simulink model "QAM16_adalm_radio_emulation"  (R2024b)
settings: Solver=VariableStepAuto  StartTime=0.0  StopTime=38  RelTol=1e-3
PreLoadFcn:
  | % 16-QAM demo. SJSU. Fall 2020
  | 
  | alpha = 1/2;
  | 
  | Rs = 400000;                     % Sampling rate for radios
  | Nf = 2000;                        % Frame size
  | 
  | Gt = -5;                             % Transmitter radio gain
  | amp = 0.5;                        % Transmited signal amplitude
  | 
  | Gr = 25;                             % Receiver radio gain
  | 
  | Deltaf = 500;                     % Frequency error
  | phi = -pi/6;                        % Phase error
  | 
  | EsNo = 20;
  | var = 10^-(EsNo/10)/2;                   % AWGN power
  | 
  | BarkerCode=[1,1,1,1,1,-1,-1,1,1,-1,1,-1,1];
  | 
  | load(QPSK_radio_parameters.mat)
PostLoadFcn:
  | laod(QPSK_radio_parameters.mat)
undefined symbols (not defined in the file or in its folder): QAM, sdrqpskrx
libraries: commrflib2 x3, commrfcorlib x2, commsync2 x2, commfilt2 x2, simulink x2, dspstat3 x1, commrandsrc3 x1, dspsigops x1, commsequence2 x1, commdigbbndam3 x1
settings Model: Creator=The MathWorks, Inc.  LastModifiedBy=14083
settings SolverCC: AlgebraicLoopSolver=TrustRegion  AutoInsertRateTranBlk=on
settings DataIOCC: LimitDataPoints=on  SaveFormat=Structure  SaveOutput=off  SignalLogging=off  DSMLogging=off  SaveTime=off  ReturnWorkspaceOutputs=off
settings OptimizationCC: DefaultParameterBehavior=Inlined  ExpressionDepthLimit=2147483647  LocalBlockOutputs=off  LifeSpan=inf  SimCompilerOptimization=on
settings DebuggingCC: AlgebraicLoopMsg=error  UnderspecifiedInitializationDetection=Classic  MergeDetectMultiDrivingBlocksExec=none  SolverPrmCheckMsg=warning  SingleTaskRateTransMsg=error  ParameterPrecisionLossMsg=none  FcnCallInpInsideContextMsg=warning  UnconnectedInputMsg=warning  UnconnectedOutputMsg=warning  UnconnectedLineMsg=warning  AllowSymbolicDim=off  StateNameClashWarn=warning  SFUnexpectedBacktrackingDiag=warning  SFNoUnconditionalDefaultTransitionDiag=warning  SFExecutionAtInitializationDiag=none  ArithmeticOperatorsInVariantConditions=warning
settings HardwareCC: ProdBitPerPointer=32  ProdBitPerSizeT=32  ProdBitPerPtrDiffT=32  ProdLargestAtomicFloat=None  ProdIntDivRoundTo=Undefined  ProdEndianess=Unspecified  ProdWordSize=32  ProdHWDeviceType=32-bit Generic  TargetBitPerPointer=64  TargetBitPerSizeT=64  TargetBitPerPtrDiffT=64  TargetLongLongMode=on  TargetIntDivRoundTo=Zero  TargetEndianess=LittleEndian  TargetWordSize=64  TargetHWDeviceType=Generic->MATLAB Host Computer  ProdEqTarget=off
settings ModelReferenceCC: EnableRefExpFcnMdlSchedulingChecks=on  PropagateSignalLabelsOutOfModel=off
settings SFSimCC: SimUseLocalCustomCode=off  CustomCodeUndefinedFunction=UseInterfaceOnly
settings RTWCC: RTWUseLocalCustomCode=off  GPUComputeCapability=3.5
settings RTWCC: CustomSourceCode=|
  | #include <stdio.h>
  | #include <stdlib.h>
settings CodeAppCC: StateflowObjectComments=on
settings GRTTargetCC: TargetLangStandard=C89/C90 (ANSI)  CombineOutputUpdateFcns=off  GRTInterface=on
settings ConfigComp: CovMetricSettings=dw  CovSaveCumulativeToWorkspaceVar=on  CovSaveSingleToWorkspaceVar=on  CovExternalEMLEnable=off  CovSFcnEnable=off

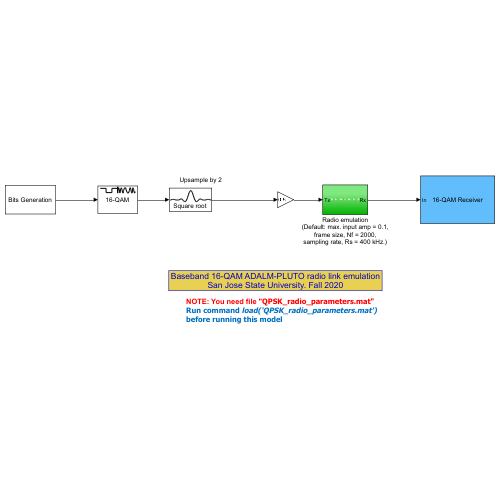
[thumbnail: Simulink's stored preview of the top-level diagram]
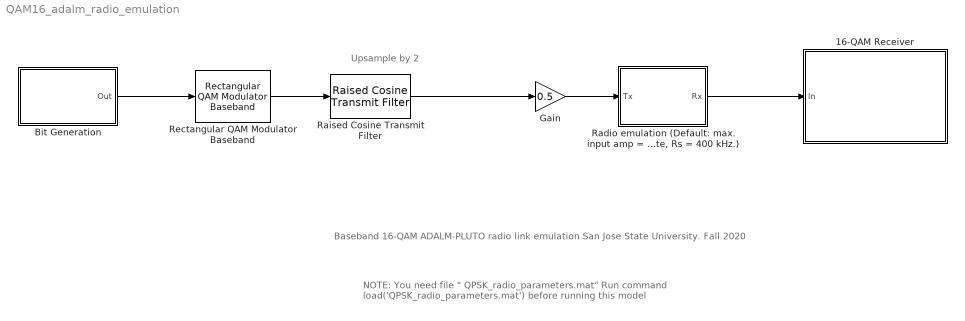
== system QAM16_adalm_radio_emulation ==
  note: NOTE: You need file " QPSK_radio_parameters.mat"
      | Run command load('QPSK_radio_parameters.mat') before running this model
  note: Upsample by 2
  note: Baseband 16-QAM ADALM-PLUTO radio link emulation
      | San Jose State University. Fall 2020
  16-QAM Receiver : Subsystem
      mask Display: disp('16-QAM Receiver')
  Bit Generation : Subsystem
      mask Display: disp('Bits Generation')
  Gain : Gain  Gain=0.5
  "Radio emulation (Default: max. input amp = 0.1, frame size, Nf = 2000, sampling rate, Rs = 400 kHz.)" : Subsystem
  Raised Cosine Transmit Filter : commfilt2/Raised Cosine Transmit Filter  filtType=Square root  R=alpha  filtSpan=10  N=2  filterGain=1  InputProcessing=Columns as channels (frame based)  RateOptions=Enforce single-rate processing  framing=Mute  checkCoeff=off  variableName=rcTxFilt1  checkGain=Normalized  sampMode=Mute  saveAsFlag=0  currentFiltSpan=10  D=5  launchFVT=on  roundingMode=Floor  overflowMode=off  coeffDataTypeStr=Inherit: Same word length as input  coeffMin=[]  coeffMax=[]  coeffLastDataTypeStr=Inherit: Same word length as input  outputDataTypeStr=Inherit: Same as accumulator  outputMin=[]  outputMax=[]  outputLastDataTypeStr=Inherit: Same as accumulator
  Rectangular QAM Modulator Baseband : commdigbbndam3/Rectangular QAM Modulator Baseband  M=16  InType=Bit  Enc=Gray  Mapping=[0:15]  PowType=Average Power  MinDist=2  AvgPow=1  PeakPow=1  Ph=0  outDtype=double  outWordLen=16  outUDDataType=sfix(16)  outFracLenMode=Best precision  outFracLen=15  outDataTypeStr=double  outLastDataTypeStr=double
  wires:
  Bit Generation/1(Out) -> Rectangular QAM Modulator Baseband/1
  "Radio emulation (Default: max. input amp = 0.1, frame size, Nf = 2000, sampling rate, Rs = 400 kHz.)"/1(Rx) -> 16-QAM Receiver/1(In)
  Rectangular QAM Modulator Baseband/1 -> Raised Cosine Transmit Filter/1
  Gain/1 -> "Radio emulation (Default: max. input amp = 0.1, frame size, Nf = 2000, sampling rate, Rs = 400 kHz.)"/1(Tx)
  Raised Cosine Transmit Filter/1 -> Gain/1

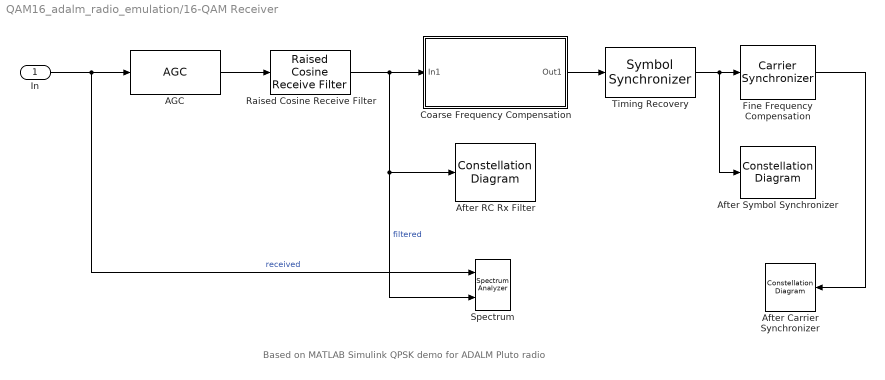
== system QAM16_adalm_radio_emulation/16-QAM Receiver ==
  note: Based on MATLAB Simulink QPSK demo for ADALM Pluto radio
  In : Inport
  AGC : commrfcorlib/AGC  LegacyMode=off  DetectorMethod=Rectifier  LoopMethod=Linear  UpdatePeriod=100  StepSize=0.1  AdaptationStepSize=0.01  DesiredOutputPower=1  AveragingLength=sdrqpskrx.AveragingLength  MaximumGain=30  MaxPowerGain=sdrqpskrx.MaxPowerGain  GainOutputPort=off  InputPowerOutputPort=off  SimulateUsing=Code generation
  After Carrier Synchronizer : ConstellationDiagram  Tag=ScatterPlot  WindowPosition=[1063.000000,378.000000,414.000000,420.000000,]  Visible=on  ScopeFrameLocation=window  SamplesPerSymbol=sdrqpskrx.Interpolation  SymbolsToDisplaySource=Property  SymbolsToDisplay=sdrqpskrx.FrameSize  ReferenceConstellation=16-QAM  Title=After Carrier Synchronizer  XLimits=[-3.25,3.25]  YLimits=[-2.8 2.8]  ShowReferenceConstellation=off  ColorFading=on  DefaultConfigurationName=comm.scopes.ConstellationDiagramBlockCfg
  After RC Rx Filter : ConstellationDiagram  Tag=ScatterPlot  WindowPosition=[218.000000,376.000000,414.000000,423.000000,]  Visible=on  ScopeFrameLocation=window  SamplesPerSymbol=sdrqpskrx.Interpolation  SymbolsToDisplaySource=Property  SymbolsToDisplay=sdrqpskrx.FrameSize  ReferenceConstellation=16-QAM  Title=After Raised Cosine Rx Filter  XLimits=[-2.6623352812286596,2.6684400675627136]  YLimits=[-2.6508250238276854,2.7130991397079955]  ShowReferenceConstellation=off  ColorFading=on  DefaultConfigurationName=comm.scopes.ConstellationDiagramBlockCfg
  After Symbol Synchronizer : ConstellationDiagram  Tag=ScatterPlot  WindowPosition=[633.000000,376.000000,432.000000,422.000000,]  Visible=on  ScopeFrameLocation=window  SamplesPerSymbol=2  SymbolsToDisplaySource=Property  SymbolsToDisplay=sdrqpskrx.FrameSize  ReferenceConstellation=QPSK  Title=After Symbol Synchronizer  XLimits=[-3.4,3.4]  YLimits=[-2.8 2.8]  ShowReferenceConstellation=off  ColorFading=on  DefaultConfigurationName=comm.scopes.ConstellationDiagramBlockCfg
  Coarse Frequency Compensation : Subsystem
      mask Display: fprintf('Coarse Frequency\nCompensation')
  Fine Frequency Compensation : commsync2/Carrier Synchronizer  Modulation=QAM  ModulationPhaseOffset=Auto  CustomPhaseOffset=0  SamplesPerSymbol=sdrqpskrx.Interpolation/sdrqpskrx.Decimation  DampingFactor=1  NormalizedLoopBandwidth=0.01  EstimatedPhaseErrorOutputPort=off  SimulateUsing=Code generation
  Raised Cosine Receive Filter : commfilt2/Raised Cosine Receive Filter  filtType=Square root  R=alpha  filtSpan=sdrqpskrx.RaisedCosineFilterSpan  N=sdrqpskrx.Interpolation  downFactor=sdrqpskrx.Decimation  downOffset=0  filterGain=1  InputProcessing=Columns as channels (frame based)  RateOptions=Enforce single-rate processing  framing=Mute  checkCoeff=off  variableName=rcRxFilt  currentFiltSpan=10  D=5  inputOffset=0  sampMode=Mute  saveAsFlag=0  rateMode=Downsampling  checkGain=Normalized  launchFVT=on  roundingMode=Floor  overflowMode=off  coeffDataTypeStr=Inherit: Same word length as input  coeffMin=[]  coeffMax=[]  coeffLastDataTypeStr=Inherit: Same word length as input  accumDataTypeStr=Inherit: Same as product output  accumLastDataTypeStr=Inherit: Same as product output  outputDataTypeStr=Inherit: Same as accumulator  outputMin=[]  outputMax=[]  outputLastDataTypeStr=Inherit: Same as accumulator
  Spectrum : SpectrumAnalyzer  NumInputPorts=2  WindowPosition=[27.000000,20.000000,800.000000,364.000000,]  Visible=on  ScopeFrameLocation=window  Method=Welch  SampleRate=100654.15132949  AxesScaling=Manual  RBWSource=Property  RBW=75  FFTLength=128  Span=100000  StartFrequency=-50000  StopFrequency=50000  AveragingMethod=Running  SpectralAverages=2  SpectrumUnits=dBW  Title=Before and After Raised Cosine Rx Filter  YLabel=Power Spectrum  YLimits=[-137.6344738236879266,40]  ShowLegend=on  AllowFFTLengthLessThanSamplesPerUpdate=on  DefaultConfigurationName=spbscopes.SpectrumAnalyzerBlockCfg  IsFrequencyInputMode=0  FrequencyVectorPort=0  FrequencyVectorFromPort=0  FrequencyInputRBWPort=0  FrequencyInputRBWFromPort=0
  Timing Recovery : commsync2/Symbol Synchronizer  Modulation=PAM/PSK/QAM  TimingErrorDetector=Gardner (non-data-aided)  SamplesPerSymbol=sdrqpskrx.Interpolation/sdrqpskrx.Decimation  DampingFactor=1  NormalizedLoopBandwidth=0.01  DetectorGain=sdrqpskrx.TimingErrorDetectorGain  TimingErrorOutputPort=off  SimulateUsing=Code generation
  wires:
  Raised Cosine Receive Filter/1 -> Coarse Frequency Compensation/1(In1), Spectrum/2, After RC Rx Filter/1  "filtered"
  Coarse Frequency Compensation/1(Out1) -> Timing Recovery/1
  AGC/1 -> Raised Cosine Receive Filter/1
  Fine Frequency Compensation/1 -> After Carrier Synchronizer/1
  Timing Recovery/1 -> Fine Frequency Compensation/1, After Symbol Synchronizer/1
  In/1 -> Spectrum/1, AGC/1  "received"

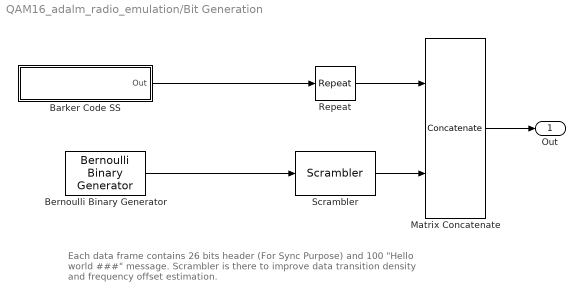
== system QAM16_adalm_radio_emulation/Bit Generation ==
  note: Each data frame contains 26 bits header (For Sync Purpose) and 100
      | "Hello world ###" message. Scrambler is there to improve data
      | transition density and frequency offset estimation.
  Barker Code SS : Subsystem
      mask Display: disp('Unipolar\nBarker Code')
  Bernoulli Binary Generator : commrandsrc3/Bernoulli Binary Generator  ProbabilityOfZero=0.5  SeedSource=Auto  Seed=0  SampleTime=1/200000  SamplesPerFrame=100*40-13*2  OutputDataType=double  SimulateUsing=Interpreted execution
  Matrix Concatenate : Concatenate  Mode=Multidimensional array
  Repeat : dspsigops/Repeat  FactorSource=Dialog parameter  N=2  Nmax=16  InputProcessing=Columns as channels (frame based)  RateOptions=Enforce single-rate processing  ic=0  mode=Unused parameter value
  Scrambler : commsequence2/Scrambler  M=2  poly=[1 1 1 0 1]  iniStaSource=Dialog Parameter  ini_sta=[0 0 0 0]  resetViaPort=off
  Out : Outport  VectorParamsAs1DForOutWhenUnconnected=off
  wires:
  Barker Code SS/1(Out) -> Repeat/1
  Matrix Concatenate/1 -> Out/1
  Repeat/1 -> Matrix Concatenate/1
  Scrambler/1 -> Matrix Concatenate/2
  Bernoulli Binary Generator/1 -> Scrambler/1

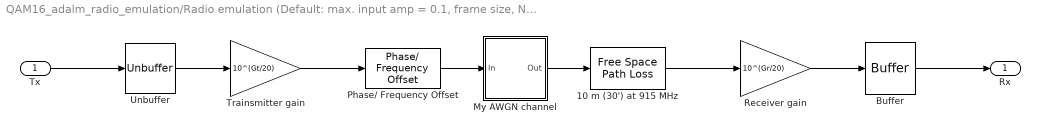
== system QAM16_adalm_radio_emulation/Radio emulation (Default: max. input amp = 0.1, frame size, Nf = 2000, sampling rate, Rs = 400 kHz.) ==
  Tx : Inport
  10 m (30') at 915 MHz : commrflib2/Free Space Path Loss  mode=Distance and Frequency  dB=10  d=10/1000  fc=915
  Buffer : Buffer  N=Nf  OutputFrames=off
  My AWGN channel : Subsystem
  Phase/ Frequency Offset : commrflib2/Phase// Frequency Offset  phaseOffset=phi  freqPort=off  freqOffset=Deltaf
  Receiver gain : Gain  Gain=10^(Gr/20)
  Trainsmitter gain : Gain  Gain=10^(Gt/20)
  Unbuffer : Unbuffer
  Rx : Outport
  wires:
  Tx/1 -> Unbuffer/1
  My AWGN channel/1(Out) -> 10 m (30') at 915 MHz/1
  Phase/ Frequency Offset/1 -> My AWGN channel/1(In)
  10 m (30') at 915 MHz/1 -> Receiver gain/1
  Receiver gain/1 -> Buffer/1
  Unbuffer/1 -> Trainsmitter gain/1
  Buffer/1 -> Rx/1
  Trainsmitter gain/1 -> Phase/ Frequency Offset/1

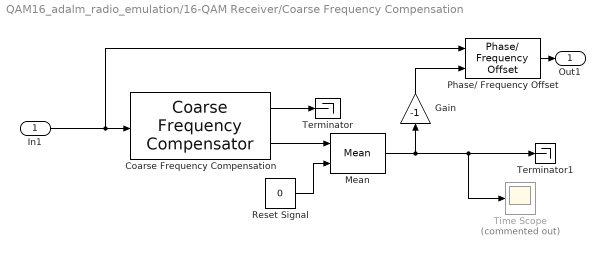
== system QAM16_adalm_radio_emulation/16-QAM Receiver/Coarse Frequency Compensation ==
  In1 : Inport
  Coarse Frequency Compensation : commrfcorlib/Coarse Frequency Compensator  Modulation=QPSK  Algorithm=Correlation-based  FrequencyResolution=25  MaximumFrequencyOffset=12.5e3  SamplesPerSymbol=4  EstimatedFreqOffsetPort=on  SimulateUsing=Code generation
  Gain : Gain  Gain=-1
  Mean : dspstat3/Mean  run=on  InputProcessing=Columns as channels (frame based)  reset_popup=Either edge  directionMode=Each column  dimension=1  roiEnable=off  roiType=Rectangles  roiPortion=Entire ROI  roiOutput=Individual statistics for each ROI  roiFlag=off  roundingMode=Floor  overflowMode=off  outputDataTypeStr=Inherit: Same as accumulator  outputMin=[]  outputMax=[]  outputLastDataTypeStr=Inherit: Same as accumulator
  Phase/ Frequency Offset : commrflib2/Phase// Frequency Offset  phaseOffset=0  freqPort=on  freqOffset=0
  Reset Signal : Constant  Value=0
  Terminator : Terminator
  Terminator1 : Terminator
  Time Scope : Scope  Commented=on
  Out1 : Outport  VectorParamsAs1DForOutWhenUnconnected=off
  wires:
  In1/1 -> Phase/ Frequency Offset/1, Coarse Frequency Compensation/1
  Phase/ Frequency Offset/1 -> Out1/1
  Mean/1 -> Time Scope/1, Terminator1/1, Gain/1
  Coarse Frequency Compensation/2 -> Mean/1
  Coarse Frequency Compensation/1 -> Terminator/1
  Gain/1 -> Phase/ Frequency Offset/2
  Reset Signal/1 -> Mean/2

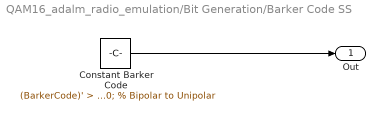
== system QAM16_adalm_radio_emulation/Bit Generation/Barker Code SS ==
  Constant Barker Code : Constant  Value=(BarkerCode)' > 0; % Bipolar to Unipolar  VectorParams1D=off  OutDataTypeStr=double
  Out : Outport  VectorParamsAs1DForOutWhenUnconnected=off
  wires:
  Constant Barker Code/1 -> Out/1

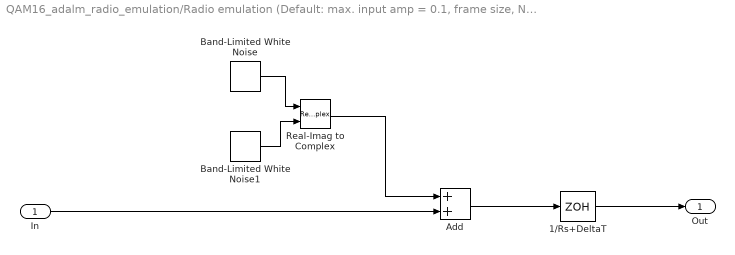
== system QAM16_adalm_radio_emulation/Radio emulation (Default: max. input amp = 0.1, frame size, Nf = 2000, sampling rate, Rs = 400 kHz.)/My AWGN channel ==
  In : Inport
  1/Rs+DeltaT : ZeroOrderHold  SampleTime=3.974/Rs+1e-11
  Add : Sum
  Band-Limited White Noise : simulink/Sources/Band-Limited White Noise  Cov=[10^(Gt/10)*var/Rs]  Ts=3.974/Rs  seed=[23341]
  Band-Limited White Noise1 : simulink/Sources/Band-Limited White Noise  Cov=[10^(Gt/10)*var/Rs]  Ts=3.974/Rs  seed=[12345]
  Real-Imag to Complex : RealImagToComplex
  Out : Outport
  wires:
  Add/1 -> 1/Rs+DeltaT/1
  Band-Limited White Noise/1 -> Real-Imag to Complex/1
  Band-Limited White Noise1/1 -> Real-Imag to Complex/2
  Real-Imag to Complex/1 -> Add/1
  1/Rs+DeltaT/1 -> Out/1
  In/1 -> Add/2
